simulink model "quad_quaternion_tracking"  (R2025b)
settings: Solver=VariableStepAuto  StartTime=0.0  StopTime=10.0  RelTol=1e-3
StopFcn:
  | quad_animation
undefined symbols (not defined in the file): g, J, m, omega0, q0_init, xi0, xidot0
settings Model: Creator=ASUS  LastModifiedBy=ASUS

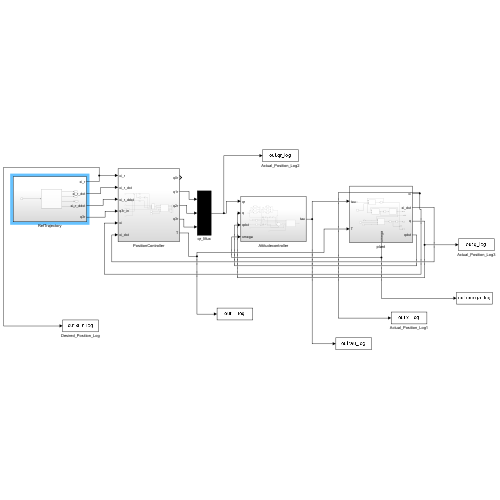
[thumbnail: Simulink's stored preview of the top-level diagram]
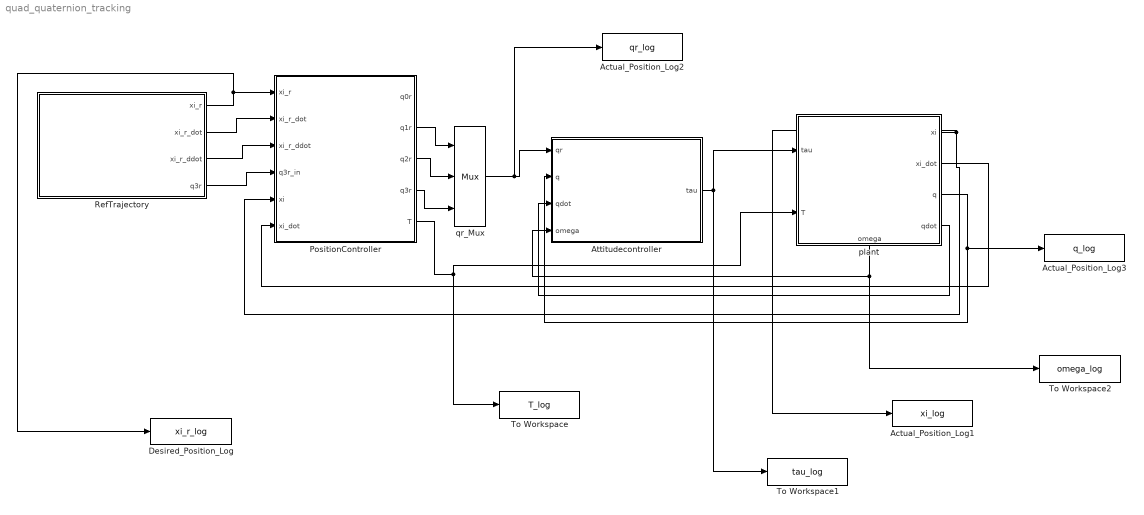
== system quad_quaternion_tracking ==
  Actual_Position_Log1 : ToWorkspace  VariableName=xi_log  SaveFormat=Timeseries  SampleTime=-1
  Actual_Position_Log2 : ToWorkspace  VariableName=qr_log  SaveFormat=Timeseries  SampleTime=-1
  Actual_Position_Log3 : ToWorkspace  VariableName=q_log  SaveFormat=Timeseries  SampleTime=-1
  Attitudecontroller : Subsystem
  Desired_Position_Log : ToWorkspace  VariableName=xi_r_log  SaveFormat=Timeseries  SampleTime=-1
  PositionController : Subsystem
  RefTrajectory : Subsystem
  To Workspace : ToWorkspace  VariableName=T_log  SaveFormat=Timeseries  SampleTime=-1
  To Workspace1 : ToWorkspace  VariableName=tau_log  SaveFormat=Timeseries  SampleTime=-1
  To Workspace2 : ToWorkspace  VariableName=omega_log  SaveFormat=Timeseries  SampleTime=-1
  plant : Subsystem
      settings: PortSchema="{\"entries\":[{\"content\":{\"sides\":[{\"content\":{\"connectorIds\":[\"In1\",\"In2\"]},\"type\":\"ConnectorPlacement.EquallySpacedRectSide\",\"uuid\":\"daf98077-7c24-429b-ae6f-25788d622914\"},{\"content\":{\"connectorIds\":[\"Out1\",\"Out2\",\"Out3\",\"Out4\"],\"side\":\"RIGHT\"},\"type\":\"ConnectorPlacement.EquallySpacedRectSide\",\"uuid\":\"3fd00f15-8adb-4cea-8a6f-ff5caff419f1\"},{\"content\":{\"side\":\"TOP\"},\"type\":\"ConnectorPlacement.EquallySpacedRectSide\",\"uuid\":\"bc39026f-8ae5-435d-80aa-ac75e1f966dc\"},{\"content\":{\"connectorIds\":[\"Out5\"],\"side\":\"BOTTOM\"},\"type\":\"ConnectorPlacement.EquallySpacedRectSide\",\"uuid\":\"f2d81a6b-272d-405c-bcc2-73243a95cee4\"}]},\"type\":\"ConnectorPlacement.EquallySpacedConnector\",\"uuid\":\"f47e6c5f-8c09-48f0-90bc-b2c9317e6b42\"}],\"packageUris\":[\"http://schema.mathworks.com/mf0/Connector/R2020b\"],\"version\":\"1.0\"}"
  qr_Mux : Mux  Inputs=3
  wires:
  RefTrajectory/1(xi_r) -> Desired_Position_Log/1, PositionController/1(xi_r)
  RefTrajectory/2(xi_r_dot) -> PositionController/2(xi_r_dot)
  RefTrajectory/3(xi_r_ddot) -> PositionController/3(xi_r_ddot)
  RefTrajectory/4(q3r) -> PositionController/4(q3r_in)
  plant/2(xi_dot) -> PositionController/6(xi_dot)
  PositionController/2(q1r) -> qr_Mux/1
  PositionController/3(q2r) -> qr_Mux/2
  PositionController/4(q3r) -> qr_Mux/3
  qr_Mux/1 -> Actual_Position_Log2/1, Attitudecontroller/1(qr)
  plant/4(qdot) -> Attitudecontroller/3(qdot)
  plant/5(omega) -> To Workspace2/1, Attitudecontroller/4(omega)
  Attitudecontroller/1(tau) -> To Workspace1/1, plant/1(tau)
  PositionController/5(T) -> To Workspace/1, plant/2(T)
  plant/1(xi) -> PositionController/5(xi), Actual_Position_Log1/1
  plant/3(q) -> Actual_Position_Log3/1, Attitudecontroller/2(q)

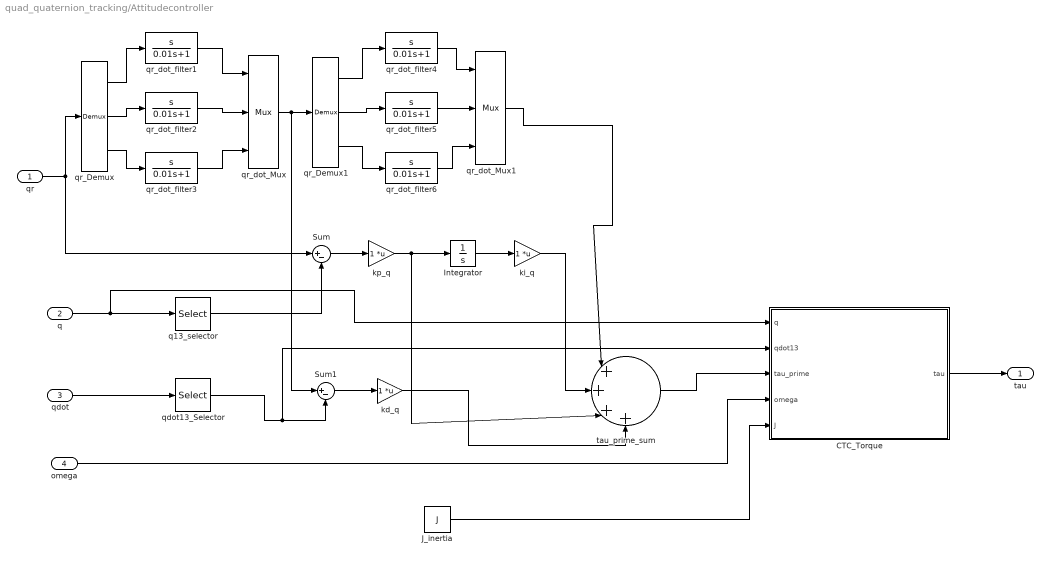
== system quad_quaternion_tracking/Attitudecontroller ==
  qr : Inport
  q : Inport  Port=2
  qdot : Inport  Port=3
  omega : Inport  Port=4
  CTC_Torque : MATLAB Function  TreatAsAtomicUnit=on
  Integrator : Integrator
  J_inertia : Constant  Value=J
  Sum : Sum  Inputs=|+-
  Sum1 : Sum  Inputs=|+-
  kd_q : Gain  Multiplication=Matrix(K*u)
  ki_q : Gain  Multiplication=Matrix(K*u)
  "kp_q " : Gain  Multiplication=Matrix(K*u)
  q13_selector : Selector  InputPortWidth=4  IndexOptions=Index vector (dialog)  Indices=[2:4]  OutputSizes=1
  qdot13_Selector : Selector  InputPortWidth=4  IndexOptions=Index vector (dialog)  Indices=[2:4]  OutputSizes=1
  qr_Demux : Demux  Outputs=3
  qr_Demux1 : Demux  Outputs=3
  qr_dot_Mux : Mux  Inputs=3
  qr_dot_Mux1 : Mux  Inputs=3
  qr_dot_filter{1..6} (6 alike) : TransferFcn  Numerator=[1 0]  Denominator=[0.01 1]
  tau_prime_sum : Sum  Inputs=|++++
  tau : Outport  VectorParamsAs1DForOutWhenUnconnected=off
  wires:
  qr/1 -> qr_Demux/1, Sum/1
  q/1 -> CTC_Torque/1(q), q13_selector/1
  Sum/1 -> "kp_q "/1
  q13_selector/1 -> Sum/2
  Integrator/1 -> ki_q/1
  qdot/1 -> qdot13_Selector/1
  qdot13_Selector/1 -> CTC_Torque/2(qdot13), Sum1/2
  Sum1/1 -> kd_q/1
  qr_dot_Mux1/1 -> tau_prime_sum/1
  ki_q/1 -> tau_prime_sum/2
  "kp_q "/1 -> tau_prime_sum/3, Integrator/1
  kd_q/1 -> tau_prime_sum/4
  tau_prime_sum/1 -> CTC_Torque/3(tau_prime)
  omega/1 -> CTC_Torque/4(omega)
  J_inertia/1 -> CTC_Torque/5(J)
  CTC_Torque/1(tau) -> tau/1
  qr_Demux/1 -> qr_dot_filter1/1
  qr_Demux/2 -> qr_dot_filter2/1
  qr_Demux/3 -> qr_dot_filter3/1
  qr_dot_filter1/1 -> qr_dot_Mux/1
  qr_dot_filter2/1 -> qr_dot_Mux/2
  qr_dot_filter3/1 -> qr_dot_Mux/3
  qr_dot_Mux/1 -> Sum1/1, qr_Demux1/1
  qr_Demux1/1 -> qr_dot_filter4/1
  qr_Demux1/2 -> qr_dot_filter5/1
  qr_Demux1/3 -> qr_dot_filter6/1
  qr_dot_filter4/1 -> qr_dot_Mux1/1
  qr_dot_filter5/1 -> qr_dot_Mux1/2
  qr_dot_filter6/1 -> qr_dot_Mux1/3

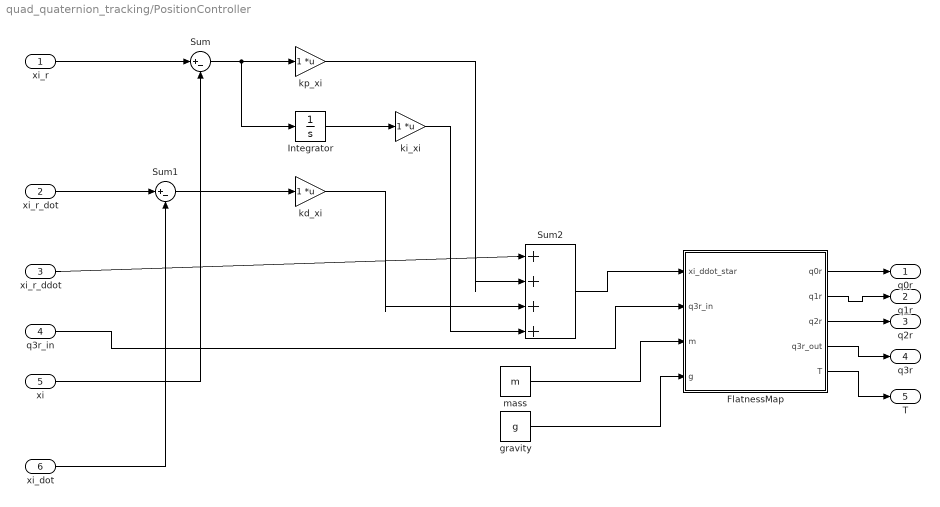
== system quad_quaternion_tracking/PositionController ==
  xi_r : Inport
  xi_r_dot : Inport  Port=2
  xi_r_ddot : Inport  Port=3
  q3r_in : Inport  Port=4
  xi : Inport  Port=5
  xi_dot : Inport  Port=6
  FlatnessMap : MATLAB Function  TreatAsAtomicUnit=on
  Integrator : Integrator
  Sum : Sum  Inputs=|+-
  Sum1 : Sum  Inputs=|+-
  Sum2 : Sum  Inputs=|++++
  gravity : Constant  Value=g
  kd_xi : Gain  Multiplication=Matrix(K*u)
  "ki_xi " : Gain  Multiplication=Matrix(K*u)
  kp_xi : Gain  Multiplication=Matrix(K*u)
  mass : Constant  Value=m
  q0r : Outport  VectorParamsAs1DForOutWhenUnconnected=off
  q1r : Outport  Port=2  VectorParamsAs1DForOutWhenUnconnected=off
  q2r : Outport  Port=3  VectorParamsAs1DForOutWhenUnconnected=off
  q3r : Outport  Port=4  VectorParamsAs1DForOutWhenUnconnected=off
  T : Outport  Port=5  VectorParamsAs1DForOutWhenUnconnected=off
  wires:
  xi_r/1 -> Sum/1
  xi/1 -> Sum/2
  Integrator/1 -> "ki_xi "/1
  kp_xi/1 -> Sum2/2
  xi_r_dot/1 -> Sum1/1
  xi_dot/1 -> Sum1/2
  Sum1/1 -> kd_xi/1
  xi_r_ddot/1 -> Sum2/1
  kd_xi/1 -> Sum2/3
  Sum/1 -> Integrator/1, kp_xi/1
  "ki_xi "/1 -> Sum2/4
  Sum2/1 -> FlatnessMap/1(xi_ddot_star)
  q3r_in/1 -> FlatnessMap/2(q3r_in)
  mass/1 -> FlatnessMap/3(m)
  gravity/1 -> FlatnessMap/4(g)
  FlatnessMap/1(q0r) -> q0r/1
  FlatnessMap/2(q1r) -> q1r/1
  FlatnessMap/3(q2r) -> q2r/1
  FlatnessMap/4(q3r_out) -> q3r/1
  FlatnessMap/5(T) -> T/1

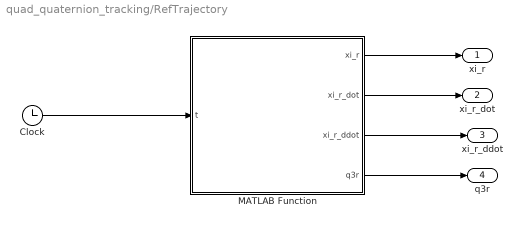
== system quad_quaternion_tracking/RefTrajectory ==
  Clock : Clock
  MATLAB Function : MATLAB Function  TreatAsAtomicUnit=on
  xi_r : Outport  VectorParamsAs1DForOutWhenUnconnected=off
  xi_r_dot : Outport  Port=2  VectorParamsAs1DForOutWhenUnconnected=off
  xi_r_ddot : Outport  Port=3  VectorParamsAs1DForOutWhenUnconnected=off
  q3r : Outport  Port=4  VectorParamsAs1DForOutWhenUnconnected=off
  wires:
  Clock/1 -> MATLAB Function/1(t)
  MATLAB Function/4(q3r) -> q3r/1
  MATLAB Function/3(xi_r_ddot) -> xi_r_ddot/1
  MATLAB Function/2(xi_r_dot) -> xi_r_dot/1
  MATLAB Function/1(xi_r) -> xi_r/1

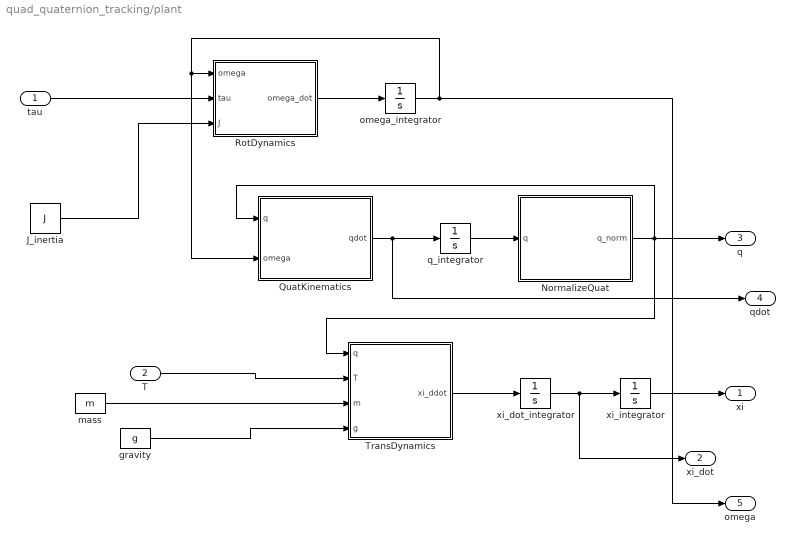
== system quad_quaternion_tracking/plant ==
  tau : Inport
  T : Inport  Port=2
  J_inertia : Constant  Value=J
  NormalizeQuat : MATLAB Function  TreatAsAtomicUnit=on
  QuatKinematics : MATLAB Function  TreatAsAtomicUnit=on
  RotDynamics : MATLAB Function  TreatAsAtomicUnit=on
  TransDynamics : MATLAB Function  TreatAsAtomicUnit=on
  gravity : Constant  Value=g
  mass : Constant  Value=m
  omega_integrator : Integrator  InitialCondition=omega0
  q_integrator : Integrator  InitialCondition=q0_init
  xi_dot_integrator : Integrator  InitialCondition=xidot0
  xi_integrator : Integrator  InitialCondition=xi0
  xi : Outport  VectorParamsAs1DForOutWhenUnconnected=off
  xi_dot : Outport  Port=2  VectorParamsAs1DForOutWhenUnconnected=off
  q : Outport  Port=3  VectorParamsAs1DForOutWhenUnconnected=off
  qdot : Outport  Port=4  VectorParamsAs1DForOutWhenUnconnected=off
  omega : Outport  Port=5  VectorParamsAs1DForOutWhenUnconnected=off
  wires:
  tau/1 -> RotDynamics/2(tau)
  J_inertia/1 -> RotDynamics/3(J)
  RotDynamics/1(omega_dot) -> omega_integrator/1
  omega_integrator/1 -> omega/1, QuatKinematics/2(omega), RotDynamics/1(omega)
  QuatKinematics/1(qdot) -> qdot/1, q_integrator/1
  q_integrator/1 -> NormalizeQuat/1(q)
  NormalizeQuat/1(q_norm) -> TransDynamics/1(q), q/1, QuatKinematics/1(q)
  T/1 -> TransDynamics/2(T)
  mass/1 -> TransDynamics/3(m)
  gravity/1 -> TransDynamics/4(g)
  TransDynamics/1(xi_ddot) -> xi_dot_integrator/1
  xi_dot_integrator/1 -> xi_dot/1, xi_integrator/1
  xi_integrator/1 -> xi/1

== matlab function quad_quaternion_tracking/RefTrajectory/MATLAB Function ==
  data: t input; xi_r output; xi_r_dot output; xi_r_ddot output; q3r output
function [xi_r, xi_r_dot, xi_r_ddot, q3r] = RefTrajectory(t)

% ============================================================
% QUINTIC REFERENCE TRAJECTORY
% Start -> Destination over complete 10 second simulation
% ============================================================

% Start position
p0 = [1.8; 2.27; 0.6];

% Destination position
p1 = [2.9; 3.0; 1.2];

% Time interval
t0 = 0;
t1 = 10;

% ------------------------------------------------------------
% Smooth trajectory from p0 to p1
% ------------------------------------------------------------

if t <= t1

    [xi_r, xi_r_dot, xi_r_ddot] = ...
        quinticSeg(t, t0, t1, p0, p1);

else

    % Hold final position after reaching destination
    xi_r = p1;
    xi_r_dot = [0;0;0];
    xi_r_ddot = [0;0;0];

end

% Desired yaw-related quaternion component
q3r = 0;

end


% ============================================================
% Quintic trajectory segment
% ============================================================

function [p,v,a] = quinticSeg(t,ta,tb,pa,pb)

T = tb-ta;

% Normalized time
tau = min(max((t-ta)/T,0),1);

% Quintic position profile
s = 10*tau.^3 ...
    - 15*tau.^4 ...
    + 6*tau.^5;

% First derivative
sd = (30*tau.^2 ...
    - 60*tau.^3 ...
    + 30*tau.^4)/T;

% Second derivative
sdd = (60*tau ...
    - 180*tau.^2 ...
    + 120*tau.^3)/T^2;

% Position
p = pa + (pb-pa).*s;

% Velocity
v = (pb-pa).*sd;

% Acceleration
a = (pb-pa).*sdd;

end

== matlab function quad_quaternion_tracking/PositionController/FlatnessMap ==
  data: xi_ddot_star input; q0r output; q3r_in input; m input; g input; q1r output; q2r output; q3r_out output; T output
function [q0r,q1r,q2r,q3r_out,T] = FlatnessMap(xi_ddot_star,q3r_in,m,g)

xdd = xi_ddot_star(1);
ydd = xi_ddot_star(2);
zdd = xi_ddot_star(3);

normA = sqrt(xdd^2 + ydd^2 + (zdd+g)^2);

T = m*normA;

q3r_out = q3r_in;

inner = (zdd+g)/normA - 2*q3r_in^2 + 1;

inner = max(inner,0);

sq = sqrt(inner);

q0r = (1/sqrt(2))*sq;

denom = (zdd+g) + normA;

denom = sign(denom)*max(abs(denom),1e-6);

q1r = (xdd*q3r_in - (1/sqrt(2))*ydd*sq)/denom;

q2r = (ydd*q3r_in + (1/sqrt(2))*xdd*sq)/denom;

end

== matlab function quad_quaternion_tracking/Attitudecontroller/CTC_Torque ==
  data: q input; tau output; qdot13 input; tau_prime input; omega input; J input
function tau = CTC_Torque(q, qdot13, tau_prime, omega, J)

Jx = J(1);
Jy = J(2);
Jz = J(3);

Jmat = diag(J);

q0 = q(1);
q1 = q(2);
q2 = q(3);
q3 = q(4);

Q = 2*[ q0  q1  q2  q3;
       -q1  q0  q3 -q2;
       -q2 -q3  q0  q1;
       -q3  q2 -q1  q0];

q0dot = -(q1*qdot13(1) + ...
          q2*qdot13(2) + ...
          q3*qdot13(3)) / max(q0,1e-6);

qdot_full = [q0dot;
             qdot13];

Qq = Q(2:4,:);

tau = Jmat*(Qq*[0;tau_prime]) ...
      + cross(omega,Jmat*omega);

end

== matlab function quad_quaternion_tracking/plant/RotDynamics ==
  data: omega input; omega_dot output; tau input; J input
function omega_dot = RotDynamics(omega,tau,J)

Jx = J(1);
Jy = J(2);
Jz = J(3);

wx = omega(1);
wy = omega(2);
wz = omega(3);

omega_dot = [
    (Jy-Jz)/Jx*wy*wz + tau(1)/Jx;
    (Jz-Jx)/Jy*wz*wx + tau(2)/Jy;
    (Jx-Jy)/Jz*wx*wy + tau(3)/Jz
];

end

== matlab function quad_quaternion_tracking/plant/QuatKinematics ==
  data: q input; qdot output; omega input
function qdot = QuatKinematics(q,omega)

q0 = q(1);
q1 = q(2);
q2 = q(3);
q3 = q(4);

wx = omega(1);
wy = omega(2);
wz = omega(3);

Omega = [
    0  -wx  -wy  -wz;
    wx  0    wz  -wy;
    wy -wz   0    wx;
    wz  wy  -wx   0
];

qdot = 0.5*Omega*q;

end

== matlab function quad_quaternion_tracking/plant/NormalizeQuat ==
  data: q input; q_norm output
function q_norm = NormalizeQuat(q)

q_norm = q / norm(q);

end

== matlab function quad_quaternion_tracking/plant/TransDynamics ==
  data: q input; xi_ddot output; T input; m input; g input
function xi_ddot = TransDynamics(q,T,m,g)

q0 = q(1);
q1 = q(2);
q2 = q(3);
q3 = q(4);

R = [1-2*(q2^2+q3^2),   2*(q1*q2-q0*q3),   2*(q0*q2+q1*q3);
     2*(q1*q2+q0*q3),   1-2*(q1^2+q3^2),   2*(q2*q3-q0*q1);
     2*(q1*q3-q0*q2),   2*(q0*q1+q2*q3),   1-2*(q1^2+q2^2)];

xi_ddot = [0;0;-g] + (T/m)*(R*[0;0;1]);

end
